simulink model "Tank_test"  (R2014b)
settings: Solver=ode23tb  StartTime=0.0  StopTime=100  RelTol=1e-3
libraries: DAEMOT_Lib x3
settings Model: Creator=pangbor2  LastModifiedBy=koeln2

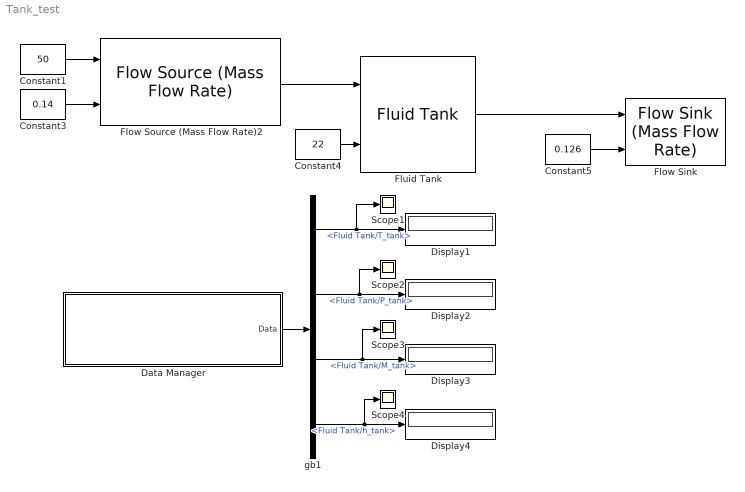
== system Tank_test ==
  Constant1 : Constant  Value=50
  Constant3 : Constant  Value=0.14
  Constant4 : Constant  Value=22
  Constant5 : Constant  Value=0.126
  Data Manager : Subsystem  AncestorBlock=DAEMOT_Lib/Support Functions/Data Manager  mask{null=0}
      mask init:
      | set_param(gcb, 'LinkStatus', 'inactive')    % disable the library link
      settings: OpenFcn=data_manager
      mask Display: str ='Fluid Tank/T_tank\nFluid Tank/P_tank\nFluid Tank/M_tank\nFluid Tank/h_tank'; fprintf(str)
  Display{1..4} (4 alike) : Display
  Flow Sink : DAEMOT_Lib/Components/Flow Sink (Mass Flow Rate)  M_ext=on  M=0  T_ext=on  T=0  P_ext=on  P=0
  Flow Source (Mass Flow Rate)2 : DAEMOT_Lib/Components/Flow Source (Mass Flow Rate)  M_ext=on  M=0  T_ext=on  T=0  P_ext=on  P=0
  Fluid Tank : DAEMOT_Lib/Components/Fluid Tank  fld=PG50  T_init=22  h_init=0.3  M_init=9.8367  P_init=104.0716  Tamb_init=22  H=0  D=0.2  Pamb=101
  Scope{1..4} (4 alike) : Scope
      Scope3 settings: SaveName=ScopeData2
      Scope4 settings: SaveName=ScopeData3
  gb1 : BusSelector  OutputSignals=Fluid Tank/T_tank,Fluid Tank/P_tank,Fluid Tank/M_tank,Fluid Tank/h_tank
  wires:
  Flow Source (Mass Flow Rate)2/1 -> Fluid Tank/1
  Constant5/1 -> Flow Sink/2
  Fluid Tank/1 -> Flow Sink/1
  Constant4/1 -> Fluid Tank/2
  Data Manager/1(Data) -> gb1/1
  gb1/1 -> Scope1/1, Display1/1  "<Fluid Tank/T_tank>"
  gb1/2 -> Scope2/1, Display2/1  "<Fluid Tank/P_tank>"
  gb1/3 -> Scope3/1, Display3/1  "<Fluid Tank/M_tank>"
  gb1/4 -> Scope4/1, Display4/1  "<Fluid Tank/h_tank>"
  Constant3/1 -> Flow Source (Mass Flow Rate)2/2
  Constant1/1 -> Flow Source (Mass Flow Rate)2/1

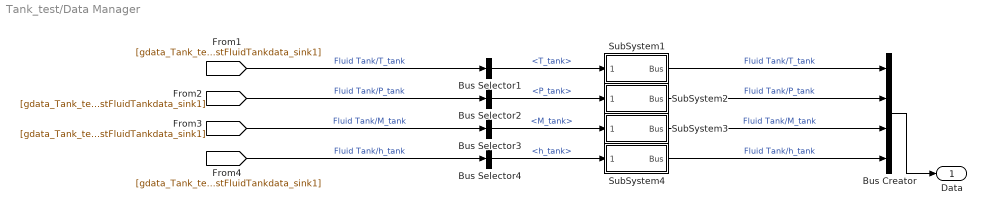
== system Tank_test/Data Manager ==
  Bus Creator : BusCreator
  Bus Selector1 : BusSelector  OutputSignals=T_tank
  Bus Selector2 : BusSelector  OutputSignals=P_tank
  Bus Selector3 : BusSelector  OutputSignals=M_tank
  Bus Selector4 : BusSelector  OutputSignals=h_tank
  SubSystem1 : Subsystem
  SubSystem2 : Subsystem
  SubSystem3 : Subsystem
  SubSystem4 : Subsystem
  Data : Outport
  wires:
  Bus Creator/1 -> Data/1
  [gdata_Tank_testFluidTankdata_sink1] -> Bus Selector1/1  "Fluid Tank/T_tank"
  Bus Selector1/1 -> SubSystem1/1(Rename)  "<T_tank>"
  SubSystem1/1(Bus) -> Bus Creator/1  "Fluid Tank/T_tank"
  [gdata_Tank_testFluidTankdata_sink1] -> Bus Selector2/1  "Fluid Tank/P_tank"
  Bus Selector2/1 -> SubSystem2/1(Rename)  "<P_tank>"
  SubSystem2/1(Bus) -> Bus Creator/2  "Fluid Tank/P_tank"
  [gdata_Tank_testFluidTankdata_sink1] -> Bus Selector3/1  "Fluid Tank/M_tank"
  Bus Selector3/1 -> SubSystem3/1(Rename)  "<M_tank>"
  SubSystem3/1(Bus) -> Bus Creator/3  "Fluid Tank/M_tank"
  [gdata_Tank_testFluidTankdata_sink1] -> Bus Selector4/1  "Fluid Tank/h_tank"
  Bus Selector4/1 -> SubSystem4/1(Rename)  "<h_tank>"
  SubSystem4/1(Bus) -> Bus Creator/4  "Fluid Tank/h_tank"

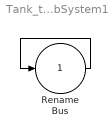
== system Tank_test/Data Manager/SubSystem1 ==
  Rename : Inport
  Bus : Outport
  wires:
  Rename/1 -> Bus/1

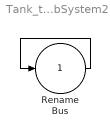
== system Tank_test/Data Manager/SubSystem2 ==
  Rename : Inport
  Bus : Outport
  wires:
  Rename/1 -> Bus/1

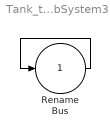
== system Tank_test/Data Manager/SubSystem3 ==
  Rename : Inport
  Bus : Outport
  wires:
  Rename/1 -> Bus/1

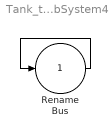
== system Tank_test/Data Manager/SubSystem4 ==
  Rename : Inport
  Bus : Outport
  wires:
  Rename/1 -> Bus/1
